simulink subsystem "Subsystem"  (R2021b)
settings: Solver=VariableStepAuto  StartTime=0.0  StopTime=10.0  RelTol=1e-3
settings Model: Creator=andre  LastModifiedBy=andre

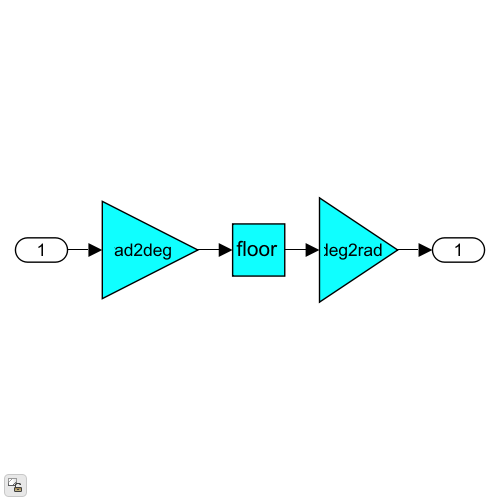
[thumbnail: Simulink's stored preview of the top-level diagram]
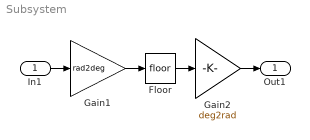
== system Subsystem ==
  In1 : Inport
  Floor : Rounding
  Gain1 : Gain  Gain=rad2deg
  Gain2 : Gain  Gain=deg2rad
  Out1 : Outport
  wires:
  In1/1 -> Gain1/1
  Floor/1 -> Gain2/1
  Gain2/1 -> Out1/1
  Gain1/1 -> Floor/1
